simulink model "prob_3"  (R2020a)
settings: Solver=VariableStepAuto  StartTime=0.0  StopTime=10.0  RelTol=1e-3
model workspace (MAT data in the model file):
  Ki = Simulink.Parameter
  Ki.Value = 40
  Ki.DataType = 'auto'
  Ki.Dimensions = [1 1]
  Kp = Simulink.Parameter
  Kp.Value = 5000
  Kp.DataType = 'auto'
  Kp.Dimensions = [1 1]
  b = Simulink.Parameter
  b.Value = 50
  b.DataType = 'auto'
  b.Dimensions = [1 1]
  m = Simulink.Parameter
  m.Value = 1000
  m.DataType = 'auto'
  m.Dimensions = [1 1]
  u = Simulink.Parameter
  u.Value = 500
  u.DataType = 'auto'
  u.Dimensions = [1 1]
settings Model: Creator=akhil singh  LastModifiedBy=akhil singh

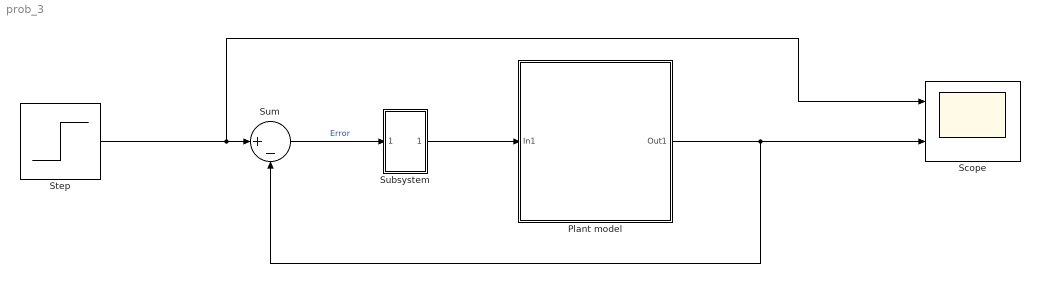
== system prob_3 ==
  Plant model : Subsystem
  Scope : Scope  NumInputPorts=2
  Step : Step  Time=0  After=u  SampleTime=0
  Subsystem : Subsystem
  Sum : Sum  Inputs=|+-
  wires:
  Step/1 -> Scope/1, Sum/1
  Plant model/1(Out1) -> Scope/2, Sum/2
  Subsystem/1(Out1) -> Plant model/1(In1)
  Sum/1 -> Subsystem/1(In1)  "Error"

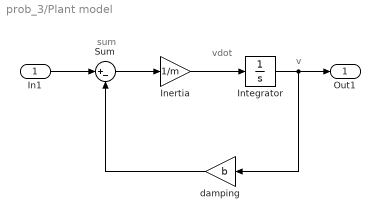
== system prob_3/Plant model ==
  note: vdot
  note: sum
  note: v
  In1 : Inport
  Inertia : Gain  Gain=1/m
  Integrator : Integrator
  Sum : Sum  Inputs=|+-
  damping : Gain  Gain=b
  Out1 : Outport
  wires:
  In1/1 -> Sum/1
  Sum/1 -> Inertia/1
  Inertia/1 -> Integrator/1
  damping/1 -> Sum/2
  Integrator/1 -> Out1/1, damping/1

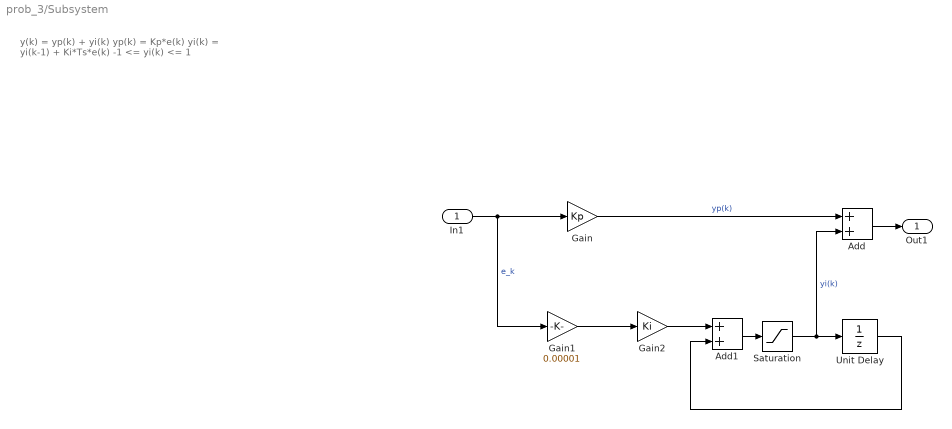
== system prob_3/Subsystem ==
  note: y(k) = yp(k) + yi(k)
      | yp(k) = Kp*e(k)
      | yi(k) = yi(k-1) + Ki*Ts*e(k)
      | -1 <= yi(k) <= 1
  In1 : Inport  OutDataTypeStr=double  PortDimensions=1  SampleTime=0
  Add : Sum
  Add1 : Sum
  Gain : Gain  Gain=Kp
  Gain1 : Gain  Gain=0.00001
  Gain2 : Gain  Gain=Ki
  Saturation : Saturate  UpperLimit=1  LowerLimit=-1
  Unit Delay : UnitDelay  SampleTime=-1  HasFrameUpgradeWarning=on
  Out1 : Outport  OutDataTypeStr=double  PortDimensions=1  SampleTime=0
  wires:
  Add/1 -> Out1/1
  Gain1/1 -> Gain2/1
  In1/1 -> Gain/1, Gain1/1  "e_k"
  Unit Delay/1 -> Add1/2
  Saturation/1 -> Unit Delay/1, Add/2  "yi(k)"
  Add1/1 -> Saturation/1
  Gain2/1 -> Add1/1
  Gain/1 -> Add/1  "yp(k)"
